simulink model "PI_control"  (R2021a)
settings: Solver=FixedStepAuto  StartTime=0.0  StopTime=10.0  RelTol=1e-3
model workspace (MAT data in the model file):
  Kp = [1131.94502275; 1488.74694893; 1864.11916894; 2165.66856904; 2408.21215527; 2770.38690321; 3112.16320972; 3434.49810271; 3512.22817626; 5299.54183511; 6428.48277688; 10024.2541154; 10535.5731133; 13219.9287748; 13082.7108791; 14529.1896787]
  Td = [1.54350351435; 1.59635610929; 1.61931871751; 1.68182843614; 1.76260260448; 1.75213760982; 1.74990764759; 1.75295644406; 1.86218984117; 2.12104616225; 2.31637617936; 1.81798900256; 1.95685563926; 1.89977500869; 2.16710938718; 2.0900037652]
  Ti = [0.0720884767012; 0.0747341757204; 0.0758835728586; 0.0790123202189; 0.0830548787748; 0.0825311515099; 0.0824195508572; 0.0825721308054; 0.0880385003906; 0.100990421055; 0.110762381868; 0.0858266289059; 0.0927754149781; 0.112767898127; 0.103294963021; 0.126587375985]
  Ts = 0.005
  v = [0.4 0.6 0.8 1 1.2 1.4 1.6 1.8 2 4 6 8 10 15 20 25]
settings Model: OrderedModelArguments=off  Creator=Henrique Mesquita  LastModifiedBy=Henrique Mesquita

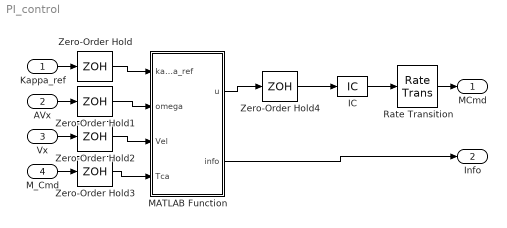
== system PI_control ==
  Kappa_ref : Inport
  AVx : Inport  Port=2
  Vx : Inport  Port=3
  M_Cmd : Inport  Port=4
  IC : InitialCondition  Value=0
  MATLAB Function : MATLAB Function  TreatAsAtomicUnit=on
  Rate Transition : RateTransition
  Zero-Order Hold{,1..4} (5 alike) : ZeroOrderHold  SampleTime=Ts
  MCmd : Outport
  Info : Outport  Port=2  OutDataTypeStr=Bus: control_info_bus
  wires:
  AVx/1 -> Zero-Order Hold1/1
  IC/1 -> Rate Transition/1
  MATLAB Function/2(info) -> Info/1
  Vx/1 -> Zero-Order Hold2/1
  M_Cmd/1 -> Zero-Order Hold3/1
  Zero-Order Hold/1 -> MATLAB Function/1(kappa_ref)
  Rate Transition/1 -> MCmd/1
  Kappa_ref/1 -> Zero-Order Hold/1
  Zero-Order Hold2/1 -> MATLAB Function/3(Vel)
  Zero-Order Hold1/1 -> MATLAB Function/2(omega)
  Zero-Order Hold4/1 -> IC/1
  Zero-Order Hold3/1 -> MATLAB Function/4(Tca)
  MATLAB Function/1(u) -> Zero-Order Hold4/1

== matlab function PI_control/MATLAB Function ==
  data: kappa_ref input; u output; omega input; Vel input; Tca input; info output Bus: control_info_bus; Kp parameter; Ti parameter; v parameter; Ts parameter; Td parameter
function [u,info] = fcn(kappa_ref, omega, Vel, Tca, Kp, Ti, v, Ts, Td)
persistent state; 
persistent ui_ant;
persistent u_ant;
persistent e_ant;

if(isempty(state) || isempty(ui_ant) || isempty(e_ant))
    state = 0;
    ui_ant = 0;
    e_ant = 0;
end

omega = omega*2*pi/60;  % rpm para rad/s
Vel = Vel/3.6;          % km/h para m/s
re = 0.284;             % raio efetivo m

% if (omega*re >= Vel)
%     kappa = (omega*re-Vel)/(omega*re+0.1);
% else
%     kappa = (omega*re-Vel)/(Vel+0.1);
% end
kappa = (omega*re-Vel)/(max([Vel 1/3.6]));
e = kappa_ref-kappa;

vsz = size(v,2);

if(Vel < (v(1)+v(2))/2)
    state = 1;
elseif(Vel < (v(vsz-1)+v(vsz))/2 && state==vsz)
    state = state - 1;
    %ui_ant = (Kp(state+1)-Kp(state))*e+(Kp(state+1)/Ti(state+1)-Kp(state)/Ti(state))*Ts/2*(e+e_ant)+ui_ant;
elseif (state < vsz)
    if(Vel > (v(state)+v(state+1))/2)
        state = state + 1;
        %ui_ant = (Kp(state-1)-Kp(state))*e+(Kp(state-1)/Ti(state-1)-Kp(state)/Ti(state))*Ts/2*(e+e_ant)+ui_ant;
    elseif(Vel < (v(state-1)+v(state))/2)
        state = state - 1;
        %ui_ant = (Kp(state+1)-Kp(state))*e+(Kp(state+1)/Ti(state+1)-Kp(state)/Ti(state))*Ts/2*(e+e_ant)+ui_ant;
    end
end
K = Kp(state); Ki = Kp(state)/Ti(state); Kd = Kp(state)*Td(state);

if(abs(Ki*Ts*(e+e_ant)/2+ui_ant)>Tca)
    ui = sign(ui_ant)*Tca;
else
    ui = Ki*Ts*(e+e_ant)/2+ui_ant;
end

ud = Kd * (e-e_ant);
du = K*e + ui + ud;

if(Tca+du>Tca)
    if(ui>0)
        ui=0;
    end
    u = Tca;
elseif (Tca+du<0)
    u = 0;
else
    u = Tca+du;
end

info = struct('Phi',0,'kappa',kappa,'u',u,'du',du,'e',e,'a',0,'ui',ui,'ud',ud,'state',state);

e_ant = e; ui_ant = ui; u_ant = u;
